simulink model "walkingRobotRL3D"  (R2020b)
settings: Solver=ode23t  StartTime=0.0  StopTime=Tf  RelTol=1e-2  EnableMultiTasking=on
PreLoadFcn:
  | robotParametersRL
undefined symbols (not defined in the file): agent, ankleD_pitch_jointMAX, ankleD_pitch_jointMIN, ankleD_roll_jointMAX, ankleD_roll_jointMIN, ankleI_pitch_jointMAX, ankleI_pitch_jointMIN, ankleI_roll_jointMAX, ankleI_roll_jointMIN, getSampleTime, height_plane, hipD_pitch_jointMAX, hipD_pitch_jointMIN, hipD_roll_jointMAX, hipD_roll_jointMIN, hipI_pitch_jointMAX, hipI_pitch_jointMIN, hipI_roll_jointMAX, hipI_roll_jointMIN, init_angs_L, init_angs_R, init_height, joint_damping, joint_limit_damping, joint_limit_stiffness, joint_stiffness, kneeD_jointMAX, kneeD_jointMIN, kneeI_jointMAX, kneeI_jointMIN, lower_leg_I0, lower_leg_length, lower_leg_mass, lower_leg_x, lower_leg_y, muscle_nominal_length, p10_ankleD_roll, plane_x, plane_y, regulator_type, tau, Tf, torso_height, torso_length, torso_offset_x, torso_offset_z, torso_width, torso_x, torso_y, torso_z, Ts, upper_leg_I0, upper_leg_length, upper_leg_mass, upper_leg_x, upper_leg_y, v10_ankleD_pitch, v10_ankleD_roll, v10_ankleI_pitch, v10_ankleI_roll ... (+41)
libraries: sm_lib x222, simulink x183, nesl_utility x130, walkingRobotUtils x69, rllib x2
(part 10 of 24)

== system walkingRobotRL3D/Check if Done22/Check correct behaviour of the muscles/Subsystem1 ==
  In1 : Inport
  In2 : Inport  Port=2
  Compare To Constant : simulink/Logic and Bit Operations/Compare To Constant  relop=<=  const=v10_ankleD_pitch  OutDataTypeStr=boolean
  Compare To Constant1 : simulink/Logic and Bit Operations/Compare To Constant  relop=>=  const=v20_ankleD_pitch  OutDataTypeStr=boolean
  Compare To Constant2 : simulink/Logic and Bit Operations/Compare To Constant  relop=>=  const=v10_ankleD_pitch  OutDataTypeStr=boolean
  Compare To Constant3 : simulink/Logic and Bit Operations/Compare To Constant  relop=<=  const=v20_ankleD_pitch  OutDataTypeStr=boolean
  Logical Operator : Logic  AllPortsSameDT=off  OutDataTypeStr=boolean
  Logical Operator1 : Logic  AllPortsSameDT=off  OutDataTypeStr=boolean
  OR : Logic  Operator=OR  IconShape=distinctive  AllPortsSameDT=off  OutDataTypeStr=boolean
  Out1 : Outport
  wires:
  In2/1 -> Compare To Constant3/1, Compare To Constant1/1
  Compare To Constant/1 -> Logical Operator/1
  Compare To Constant2/1 -> Logical Operator1/1
  OR/1 -> Out1/1
  Logical Operator1/1 -> OR/2
  In1/1 -> Compare To Constant2/1, Compare To Constant/1
  Logical Operator/1 -> OR/1
  Compare To Constant1/1 -> Logical Operator/2
  Compare To Constant3/1 -> Logical Operator1/2

== system walkingRobotRL3D/Check if Done22/Check correct behaviour of the muscles/Subsystem2 ==
  In1 : Inport
  In2 : Inport  Port=2
  Compare To Constant : simulink/Logic and Bit Operations/Compare To Constant  relop=>=  const=v10_kneeD  OutDataTypeStr=boolean
  Compare To Constant1 : simulink/Logic and Bit Operations/Compare To Constant  relop=<=  const=v20_kneeD/2  OutDataTypeStr=boolean
  Compare To Constant2 : simulink/Logic and Bit Operations/Compare To Constant  relop=>=  const=v20_kneeD/2  OutDataTypeStr=boolean
  Compare To Constant3 : simulink/Logic and Bit Operations/Compare To Constant  relop=<=  const=v20_kneeD  OutDataTypeStr=boolean
  Logical Operator : Logic  AllPortsSameDT=off  OutDataTypeStr=boolean
  Logical Operator1 : Logic  AllPortsSameDT=off  OutDataTypeStr=boolean
  OR : Logic  Operator=OR  IconShape=distinctive  AllPortsSameDT=off  OutDataTypeStr=boolean
  Out1 : Outport
  wires:
  Compare To Constant/1 -> Logical Operator/1
  Compare To Constant2/1 -> Logical Operator1/1
  OR/1 -> Out1/1
  Logical Operator1/1 -> OR/2
  Logical Operator/1 -> OR/1
  Compare To Constant1/1 -> Logical Operator/2
  Compare To Constant3/1 -> Logical Operator1/2
  In1/1 -> Compare To Constant1/1, Compare To Constant/1
  In2/1 -> Compare To Constant3/1, Compare To Constant2/1

== system walkingRobotRL3D/Check if Done22/Check correct behaviour of the muscles/Subsystem3 ==
  In1 : Inport
  In2 : Inport  Port=2
  Compare To Constant : simulink/Logic and Bit Operations/Compare To Constant  relop=<=  const=v10_hipD_roll  OutDataTypeStr=boolean
  Compare To Constant1 : simulink/Logic and Bit Operations/Compare To Constant  relop=>=  const=v20_hipD_roll  OutDataTypeStr=boolean
  Compare To Constant2 : simulink/Logic and Bit Operations/Compare To Constant  relop=>=  const=v10_hipD_roll  OutDataTypeStr=boolean
  Compare To Constant3 : simulink/Logic and Bit Operations/Compare To Constant  relop=<=  const=v20_hipD_roll  OutDataTypeStr=boolean
  Logical Operator : Logic  AllPortsSameDT=off  OutDataTypeStr=boolean
  Logical Operator1 : Logic  AllPortsSameDT=off  OutDataTypeStr=boolean
  OR : Logic  Operator=OR  IconShape=distinctive  AllPortsSameDT=off  OutDataTypeStr=boolean
  Out1 : Outport
  wires:
  In2/1 -> Compare To Constant3/1, Compare To Constant1/1
  Compare To Constant/1 -> Logical Operator/1
  Compare To Constant2/1 -> Logical Operator1/1
  OR/1 -> Out1/1
  Logical Operator1/1 -> OR/2
  In1/1 -> Compare To Constant2/1, Compare To Constant/1
  Logical Operator/1 -> OR/1
  Compare To Constant1/1 -> Logical Operator/2
  Compare To Constant3/1 -> Logical Operator1/2

== system walkingRobotRL3D/Check if Done22/Check correct behaviour of the muscles/Subsystem4 ==
  In1 : Inport
  In2 : Inport  Port=2
  Compare To Constant : simulink/Logic and Bit Operations/Compare To Constant  relop=<=  const=v10_hipD_pitch  OutDataTypeStr=boolean
  Compare To Constant1 : simulink/Logic and Bit Operations/Compare To Constant  relop=>=  const=v20_hipD_pitch  OutDataTypeStr=boolean
  Compare To Constant2 : simulink/Logic and Bit Operations/Compare To Constant  relop=>=  const=v10_hipD_pitch  OutDataTypeStr=boolean
  Compare To Constant3 : simulink/Logic and Bit Operations/Compare To Constant  relop=<=  const=v20_hipD_pitch  OutDataTypeStr=boolean
  Logical Operator : Logic  AllPortsSameDT=off  OutDataTypeStr=boolean
  Logical Operator1 : Logic  AllPortsSameDT=off  OutDataTypeStr=boolean
  OR : Logic  Operator=OR  IconShape=distinctive  AllPortsSameDT=off  OutDataTypeStr=boolean
  Out1 : Outport
  wires:
  In2/1 -> Compare To Constant3/1, Compare To Constant1/1
  Compare To Constant/1 -> Logical Operator/1
  Compare To Constant2/1 -> Logical Operator1/1
  OR/1 -> Out1/1
  Logical Operator1/1 -> OR/2
  In1/1 -> Compare To Constant2/1, Compare To Constant/1
  Logical Operator/1 -> OR/1
  Compare To Constant1/1 -> Logical Operator/2
  Compare To Constant3/1 -> Logical Operator1/2

== system walkingRobotRL3D/Check if Done22/Check correct behaviour of the muscles/Subsystem5 ==
  In1 : Inport
  In2 : Inport  Port=2
  Compare To Constant : simulink/Logic and Bit Operations/Compare To Constant  relop=<=  const=v10_ankleI_roll  OutDataTypeStr=boolean
  Compare To Constant1 : simulink/Logic and Bit Operations/Compare To Constant  relop=>=  const=v20_ankleI_roll  OutDataTypeStr=boolean
  Compare To Constant2 : simulink/Logic and Bit Operations/Compare To Constant  relop=>=  const=v10_ankleI_roll  OutDataTypeStr=boolean
  Compare To Constant3 : simulink/Logic and Bit Operations/Compare To Constant  relop=<=  const=v20_ankleI_roll  OutDataTypeStr=boolean
  Logical Operator : Logic  AllPortsSameDT=off  OutDataTypeStr=boolean
  Logical Operator1 : Logic  AllPortsSameDT=off  OutDataTypeStr=boolean
  OR : Logic  Operator=OR  IconShape=distinctive  AllPortsSameDT=off  OutDataTypeStr=boolean
  Out1 : Outport
  wires:
  In2/1 -> Compare To Constant3/1, Compare To Constant1/1
  Compare To Constant/1 -> Logical Operator/1
  Compare To Constant2/1 -> Logical Operator1/1
  OR/1 -> Out1/1
  Logical Operator1/1 -> OR/2
  In1/1 -> Compare To Constant2/1, Compare To Constant/1
  Logical Operator/1 -> OR/1
  Compare To Constant1/1 -> Logical Operator/2
  Compare To Constant3/1 -> Logical Operator1/2

== system walkingRobotRL3D/Check if Done22/Check correct behaviour of the muscles/Subsystem6 ==
  In1 : Inport
  In2 : Inport  Port=2
  Compare To Constant : simulink/Logic and Bit Operations/Compare To Constant  relop=<=  const=v10_ankleI_pitch  OutDataTypeStr=boolean
  Compare To Constant1 : simulink/Logic and Bit Operations/Compare To Constant  relop=>=  const=v20_ankleI_pitch  OutDataTypeStr=boolean
  Compare To Constant2 : simulink/Logic and Bit Operations/Compare To Constant  relop=>=  const=v10_ankleI_pitch  OutDataTypeStr=boolean
  Compare To Constant3 : simulink/Logic and Bit Operations/Compare To Constant  relop=<=  const=v20_ankleI_pitch  OutDataTypeStr=boolean
  Logical Operator : Logic  AllPortsSameDT=off  OutDataTypeStr=boolean
  Logical Operator1 : Logic  AllPortsSameDT=off  OutDataTypeStr=boolean
  OR : Logic  Operator=OR  IconShape=distinctive  AllPortsSameDT=off  OutDataTypeStr=boolean
  Out1 : Outport
  wires:
  In2/1 -> Compare To Constant3/1, Compare To Constant1/1
  Compare To Constant/1 -> Logical Operator/1
  Compare To Constant2/1 -> Logical Operator1/1
  OR/1 -> Out1/1
  Logical Operator1/1 -> OR/2
  In1/1 -> Compare To Constant2/1, Compare To Constant/1
  Logical Operator/1 -> OR/1
  Compare To Constant1/1 -> Logical Operator/2
  Compare To Constant3/1 -> Logical Operator1/2

== system walkingRobotRL3D/Check if Done22/Check correct behaviour of the muscles/Subsystem7 ==
  In1 : Inport
  In2 : Inport  Port=2
  Compare To Constant : simulink/Logic and Bit Operations/Compare To Constant  relop=<=  const=v10_hipI_roll  OutDataTypeStr=boolean
  Compare To Constant1 : simulink/Logic and Bit Operations/Compare To Constant  relop=>=  const=v20_hipI_roll  OutDataTypeStr=boolean
  Compare To Constant2 : simulink/Logic and Bit Operations/Compare To Constant  relop=>=  const=v10_hipI_roll  OutDataTypeStr=boolean
  Compare To Constant3 : simulink/Logic and Bit Operations/Compare To Constant  relop=<=  const=v20_hipI_roll  OutDataTypeStr=boolean
  Logical Operator : Logic  AllPortsSameDT=off  OutDataTypeStr=boolean
  Logical Operator1 : Logic  AllPortsSameDT=off  OutDataTypeStr=boolean
  OR : Logic  Operator=OR  IconShape=distinctive  AllPortsSameDT=off  OutDataTypeStr=boolean
  Out1 : Outport
  wires:
  In2/1 -> Compare To Constant3/1, Compare To Constant1/1
  Compare To Constant/1 -> Logical Operator/1
  Compare To Constant2/1 -> Logical Operator1/1
  OR/1 -> Out1/1
  Logical Operator1/1 -> OR/2
  In1/1 -> Compare To Constant2/1, Compare To Constant/1
  Logical Operator/1 -> OR/1
  Compare To Constant1/1 -> Logical Operator/2
  Compare To Constant3/1 -> Logical Operator1/2

== system walkingRobotRL3D/Check if Done22/Check correct behaviour of the muscles/Subsystem8 ==
  In1 : Inport
  In2 : Inport  Port=2
  Compare To Constant : simulink/Logic and Bit Operations/Compare To Constant  relop=<=  const=v10_hipI_pitch  OutDataTypeStr=boolean
  Compare To Constant1 : simulink/Logic and Bit Operations/Compare To Constant  relop=>=  const=v20_hipI_pitch  OutDataTypeStr=boolean
  Compare To Constant2 : simulink/Logic and Bit Operations/Compare To Constant  relop=>=  const=v10_hipI_pitch  OutDataTypeStr=boolean
  Compare To Constant3 : simulink/Logic and Bit Operations/Compare To Constant  relop=<=  const=v20_hipI_pitch  OutDataTypeStr=boolean
  Logical Operator : Logic  AllPortsSameDT=off  OutDataTypeStr=boolean
  Logical Operator1 : Logic  AllPortsSameDT=off  OutDataTypeStr=boolean
  OR : Logic  Operator=OR  IconShape=distinctive  AllPortsSameDT=off  OutDataTypeStr=boolean
  Out1 : Outport
  wires:
  In2/1 -> Compare To Constant3/1, Compare To Constant1/1
  Compare To Constant/1 -> Logical Operator/1
  Compare To Constant2/1 -> Logical Operator1/1
  OR/1 -> Out1/1
  Logical Operator1/1 -> OR/2
  In1/1 -> Compare To Constant2/1, Compare To Constant/1
  Logical Operator/1 -> OR/1
  Compare To Constant1/1 -> Logical Operator/2
  Compare To Constant3/1 -> Logical Operator1/2

== system walkingRobotRL3D/Check if Done22/Check correct behaviour of the muscles/Subsystem9 ==
  In1 : Inport
  In2 : Inport  Port=2
  Compare To Constant : simulink/Logic and Bit Operations/Compare To Constant  relop=>=  const=v10_kneeI  OutDataTypeStr=boolean
  Compare To Constant1 : simulink/Logic and Bit Operations/Compare To Constant  relop=<=  const=v20_kneeI/2  OutDataTypeStr=boolean
  Compare To Constant2 : simulink/Logic and Bit Operations/Compare To Constant  relop=>=  const=v20_kneeI/2  OutDataTypeStr=boolean
  Compare To Constant3 : simulink/Logic and Bit Operations/Compare To Constant  relop=<=  const=v20_kneeI  OutDataTypeStr=boolean
  Logical Operator : Logic  AllPortsSameDT=off  OutDataTypeStr=boolean
  Logical Operator1 : Logic  AllPortsSameDT=off  OutDataTypeStr=boolean
  OR : Logic  Operator=OR  IconShape=distinctive  AllPortsSameDT=off  OutDataTypeStr=boolean
  Out1 : Outport
  wires:
  Compare To Constant/1 -> Logical Operator/1
  Compare To Constant2/1 -> Logical Operator1/1
  OR/1 -> Out1/1
  Logical Operator1/1 -> OR/2
  Logical Operator/1 -> OR/1
  Compare To Constant1/1 -> Logical Operator/2
  Compare To Constant3/1 -> Logical Operator1/2
  In1/1 -> Compare To Constant1/1, Compare To Constant/1
  In2/1 -> Compare To Constant3/1, Compare To Constant2/1

== system walkingRobotRL3D/Check if Done3/Check correct behaviour of the muscles/Subsystem ==
  In1 : Inport
  In2 : Inport  Port=2
  Compare To Constant : simulink/Logic and Bit Operations/Compare To Constant  relop=<=  const=v10_ankleD_roll  OutDataTypeStr=boolean
  Compare To Constant1 : simulink/Logic and Bit Operations/Compare To Constant  relop=>=  const=v20_ankleD_roll  OutDataTypeStr=boolean
  Compare To Constant2 : simulink/Logic and Bit Operations/Compare To Constant  relop=>=  const=v10_ankleD_roll  OutDataTypeStr=boolean
  Compare To Constant3 : simulink/Logic and Bit Operations/Compare To Constant  relop=<=  const=v20_ankleD_roll  OutDataTypeStr=boolean
  Logical Operator : Logic  AllPortsSameDT=off  OutDataTypeStr=boolean
  Logical Operator1 : Logic  AllPortsSameDT=off  OutDataTypeStr=boolean
  OR : Logic  Operator=OR  IconShape=distinctive  AllPortsSameDT=off  OutDataTypeStr=boolean
  Out1 : Outport
  wires:
  In2/1 -> Compare To Constant3/1, Compare To Constant1/1
  Compare To Constant/1 -> Logical Operator/1
  Compare To Constant2/1 -> Logical Operator1/1
  OR/1 -> Out1/1
  Logical Operator1/1 -> OR/2
  In1/1 -> Compare To Constant2/1, Compare To Constant/1
  Logical Operator/1 -> OR/1
  Compare To Constant1/1 -> Logical Operator/2
  Compare To Constant3/1 -> Logical Operator1/2

== system walkingRobotRL3D/Check if Done3/Check correct behaviour of the muscles/Subsystem1 ==
  In1 : Inport
  In2 : Inport  Port=2
  Compare To Constant : simulink/Logic and Bit Operations/Compare To Constant  relop=<=  const=v10_ankleD_pitch  OutDataTypeStr=boolean
  Compare To Constant1 : simulink/Logic and Bit Operations/Compare To Constant  relop=>=  const=v20_ankleD_pitch  OutDataTypeStr=boolean
  Compare To Constant2 : simulink/Logic and Bit Operations/Compare To Constant  relop=>=  const=v10_ankleD_pitch  OutDataTypeStr=boolean
  Compare To Constant3 : simulink/Logic and Bit Operations/Compare To Constant  relop=<=  const=v20_ankleD_pitch  OutDataTypeStr=boolean
  Logical Operator : Logic  AllPortsSameDT=off  OutDataTypeStr=boolean
  Logical Operator1 : Logic  AllPortsSameDT=off  OutDataTypeStr=boolean
  OR : Logic  Operator=OR  IconShape=distinctive  AllPortsSameDT=off  OutDataTypeStr=boolean
  Out1 : Outport
  wires:
  In2/1 -> Compare To Constant3/1, Compare To Constant1/1
  Compare To Constant/1 -> Logical Operator/1
  Compare To Constant2/1 -> Logical Operator1/1
  OR/1 -> Out1/1
  Logical Operator1/1 -> OR/2
  In1/1 -> Compare To Constant2/1, Compare To Constant/1
  Logical Operator/1 -> OR/1
  Compare To Constant1/1 -> Logical Operator/2
  Compare To Constant3/1 -> Logical Operator1/2

== system walkingRobotRL3D/Check if Done3/Check correct behaviour of the muscles/Subsystem2 ==
  In1 : Inport
  In2 : Inport  Port=2
  Compare To Constant : simulink/Logic and Bit Operations/Compare To Constant  relop=>=  const=v10_kneeD  OutDataTypeStr=boolean
  Compare To Constant1 : simulink/Logic and Bit Operations/Compare To Constant  relop=<=  const=v20_kneeD/2  OutDataTypeStr=boolean
  Compare To Constant2 : simulink/Logic and Bit Operations/Compare To Constant  relop=>=  const=v20_kneeD/2  OutDataTypeStr=boolean
  Compare To Constant3 : simulink/Logic and Bit Operations/Compare To Constant  relop=<=  const=v20_kneeD  OutDataTypeStr=boolean
  Logical Operator : Logic  AllPortsSameDT=off  OutDataTypeStr=boolean
  Logical Operator1 : Logic  AllPortsSameDT=off  OutDataTypeStr=boolean
  OR : Logic  Operator=OR  IconShape=distinctive  AllPortsSameDT=off  OutDataTypeStr=boolean
  Out1 : Outport
  wires:
  Compare To Constant/1 -> Logical Operator/1
  Compare To Constant2/1 -> Logical Operator1/1
  OR/1 -> Out1/1
  Logical Operator1/1 -> OR/2
  Logical Operator/1 -> OR/1
  Compare To Constant1/1 -> Logical Operator/2
  Compare To Constant3/1 -> Logical Operator1/2
  In1/1 -> Compare To Constant1/1, Compare To Constant/1
  In2/1 -> Compare To Constant3/1, Compare To Constant2/1

== system walkingRobotRL3D/Check if Done3/Check correct behaviour of the muscles/Subsystem3 ==
  In1 : Inport
  In2 : Inport  Port=2
  Compare To Constant : simulink/Logic and Bit Operations/Compare To Constant  relop=<=  const=v10_hipD_roll  OutDataTypeStr=boolean
  Compare To Constant1 : simulink/Logic and Bit Operations/Compare To Constant  relop=>=  const=v20_hipD_roll  OutDataTypeStr=boolean
  Compare To Constant2 : simulink/Logic and Bit Operations/Compare To Constant  relop=>=  const=v10_hipD_roll  OutDataTypeStr=boolean
  Compare To Constant3 : simulink/Logic and Bit Operations/Compare To Constant  relop=<=  const=v20_hipD_roll  OutDataTypeStr=boolean
  Logical Operator : Logic  AllPortsSameDT=off  OutDataTypeStr=boolean
  Logical Operator1 : Logic  AllPortsSameDT=off  OutDataTypeStr=boolean
  OR : Logic  Operator=OR  IconShape=distinctive  AllPortsSameDT=off  OutDataTypeStr=boolean
  Out1 : Outport
  wires:
  In2/1 -> Compare To Constant3/1, Compare To Constant1/1
  Compare To Constant/1 -> Logical Operator/1
  Compare To Constant2/1 -> Logical Operator1/1
  OR/1 -> Out1/1
  Logical Operator1/1 -> OR/2
  In1/1 -> Compare To Constant2/1, Compare To Constant/1
  Logical Operator/1 -> OR/1
  Compare To Constant1/1 -> Logical Operator/2
  Compare To Constant3/1 -> Logical Operator1/2

== system walkingRobotRL3D/Check if Done3/Check correct behaviour of the muscles/Subsystem4 ==
  In1 : Inport
  In2 : Inport  Port=2
  Compare To Constant : simulink/Logic and Bit Operations/Compare To Constant  relop=<=  const=v10_hipD_pitch  OutDataTypeStr=boolean
  Compare To Constant1 : simulink/Logic and Bit Operations/Compare To Constant  relop=>=  const=v20_hipD_pitch  OutDataTypeStr=boolean
  Compare To Constant2 : simulink/Logic and Bit Operations/Compare To Constant  relop=>=  const=v10_hipD_pitch  OutDataTypeStr=boolean
  Compare To Constant3 : simulink/Logic and Bit Operations/Compare To Constant  relop=<=  const=v20_hipD_pitch  OutDataTypeStr=boolean
  Logical Operator : Logic  AllPortsSameDT=off  OutDataTypeStr=boolean
  Logical Operator1 : Logic  AllPortsSameDT=off  OutDataTypeStr=boolean
  OR : Logic  Operator=OR  IconShape=distinctive  AllPortsSameDT=off  OutDataTypeStr=boolean
  Out1 : Outport
  wires:
  In2/1 -> Compare To Constant3/1, Compare To Constant1/1
  Compare To Constant/1 -> Logical Operator/1
  Compare To Constant2/1 -> Logical Operator1/1
  OR/1 -> Out1/1
  Logical Operator1/1 -> OR/2
  In1/1 -> Compare To Constant2/1, Compare To Constant/1
  Logical Operator/1 -> OR/1
  Compare To Constant1/1 -> Logical Operator/2
  Compare To Constant3/1 -> Logical Operator1/2

== system walkingRobotRL3D/Check if Done3/Check correct behaviour of the muscles/Subsystem5 ==
  In1 : Inport
  In2 : Inport  Port=2
  Compare To Constant : simulink/Logic and Bit Operations/Compare To Constant  relop=<=  const=v10_ankleI_roll  OutDataTypeStr=boolean
  Compare To Constant1 : simulink/Logic and Bit Operations/Compare To Constant  relop=>=  const=v20_ankleI_roll  OutDataTypeStr=boolean
  Compare To Constant2 : simulink/Logic and Bit Operations/Compare To Constant  relop=>=  const=v10_ankleI_roll  OutDataTypeStr=boolean
  Compare To Constant3 : simulink/Logic and Bit Operations/Compare To Constant  relop=<=  const=v20_ankleI_roll  OutDataTypeStr=boolean
  Logical Operator : Logic  AllPortsSameDT=off  OutDataTypeStr=boolean
  Logical Operator1 : Logic  AllPortsSameDT=off  OutDataTypeStr=boolean
  OR : Logic  Operator=OR  IconShape=distinctive  AllPortsSameDT=off  OutDataTypeStr=boolean
  Out1 : Outport
  wires:
  In2/1 -> Compare To Constant3/1, Compare To Constant1/1
  Compare To Constant/1 -> Logical Operator/1
  Compare To Constant2/1 -> Logical Operator1/1
  OR/1 -> Out1/1
  Logical Operator1/1 -> OR/2
  In1/1 -> Compare To Constant2/1, Compare To Constant/1
  Logical Operator/1 -> OR/1
  Compare To Constant1/1 -> Logical Operator/2
  Compare To Constant3/1 -> Logical Operator1/2

== system walkingRobotRL3D/Check if Done3/Check correct behaviour of the muscles/Subsystem6 ==
  In1 : Inport
  In2 : Inport  Port=2
  Compare To Constant : simulink/Logic and Bit Operations/Compare To Constant  relop=<=  const=v10_ankleI_pitch  OutDataTypeStr=boolean
  Compare To Constant1 : simulink/Logic and Bit Operations/Compare To Constant  relop=>=  const=v20_ankleI_pitch  OutDataTypeStr=boolean
  Compare To Constant2 : simulink/Logic and Bit Operations/Compare To Constant  relop=>=  const=v10_ankleI_pitch  OutDataTypeStr=boolean
  Compare To Constant3 : simulink/Logic and Bit Operations/Compare To Constant  relop=<=  const=v20_ankleI_pitch  OutDataTypeStr=boolean
  Logical Operator : Logic  AllPortsSameDT=off  OutDataTypeStr=boolean
  Logical Operator1 : Logic  AllPortsSameDT=off  OutDataTypeStr=boolean
  OR : Logic  Operator=OR  IconShape=distinctive  AllPortsSameDT=off  OutDataTypeStr=boolean
  Out1 : Outport
  wires:
  In2/1 -> Compare To Constant3/1, Compare To Constant1/1
  Compare To Constant/1 -> Logical Operator/1
  Compare To Constant2/1 -> Logical Operator1/1
  OR/1 -> Out1/1
  Logical Operator1/1 -> OR/2
  In1/1 -> Compare To Constant2/1, Compare To Constant/1
  Logical Operator/1 -> OR/1
  Compare To Constant1/1 -> Logical Operator/2
  Compare To Constant3/1 -> Logical Operator1/2

== system walkingRobotRL3D/Check if Done3/Check correct behaviour of the muscles/Subsystem7 ==
  In1 : Inport
  In2 : Inport  Port=2
  Compare To Constant : simulink/Logic and Bit Operations/Compare To Constant  relop=<=  const=v10_hipI_roll  OutDataTypeStr=boolean
  Compare To Constant1 : simulink/Logic and Bit Operations/Compare To Constant  relop=>=  const=v20_hipI_roll  OutDataTypeStr=boolean
  Compare To Constant2 : simulink/Logic and Bit Operations/Compare To Constant  relop=>=  const=v10_hipI_roll  OutDataTypeStr=boolean
  Compare To Constant3 : simulink/Logic and Bit Operations/Compare To Constant  relop=<=  const=v20_hipI_roll  OutDataTypeStr=boolean
  Logical Operator : Logic  AllPortsSameDT=off  OutDataTypeStr=boolean
  Logical Operator1 : Logic  AllPortsSameDT=off  OutDataTypeStr=boolean
  OR : Logic  Operator=OR  IconShape=distinctive  AllPortsSameDT=off  OutDataTypeStr=boolean
  Out1 : Outport
  wires:
  In2/1 -> Compare To Constant3/1, Compare To Constant1/1
  Compare To Constant/1 -> Logical Operator/1
  Compare To Constant2/1 -> Logical Operator1/1
  OR/1 -> Out1/1
  Logical Operator1/1 -> OR/2
  In1/1 -> Compare To Constant2/1, Compare To Constant/1
  Logical Operator/1 -> OR/1
  Compare To Constant1/1 -> Logical Operator/2
  Compare To Constant3/1 -> Logical Operator1/2

== system walkingRobotRL3D/Check if Done3/Check correct behaviour of the muscles/Subsystem8 ==
  In1 : Inport
  In2 : Inport  Port=2
  Compare To Constant : simulink/Logic and Bit Operations/Compare To Constant  relop=<=  const=v10_hipI_pitch  OutDataTypeStr=boolean
  Compare To Constant1 : simulink/Logic and Bit Operations/Compare To Constant  relop=>=  const=v20_hipI_pitch  OutDataTypeStr=boolean
  Compare To Constant2 : simulink/Logic and Bit Operations/Compare To Constant  relop=>=  const=v10_hipI_pitch  OutDataTypeStr=boolean
  Compare To Constant3 : simulink/Logic and Bit Operations/Compare To Constant  relop=<=  const=v20_hipI_pitch  OutDataTypeStr=boolean
  Logical Operator : Logic  AllPortsSameDT=off  OutDataTypeStr=boolean
  Logical Operator1 : Logic  AllPortsSameDT=off  OutDataTypeStr=boolean
  OR : Logic  Operator=OR  IconShape=distinctive  AllPortsSameDT=off  OutDataTypeStr=boolean
  Out1 : Outport
  wires:
  In2/1 -> Compare To Constant3/1, Compare To Constant1/1
  Compare To Constant/1 -> Logical Operator/1
  Compare To Constant2/1 -> Logical Operator1/1
  OR/1 -> Out1/1
  Logical Operator1/1 -> OR/2
  In1/1 -> Compare To Constant2/1, Compare To Constant/1
  Logical Operator/1 -> OR/1
  Compare To Constant1/1 -> Logical Operator/2
  Compare To Constant3/1 -> Logical Operator1/2

== system walkingRobotRL3D/Check if Done3/Check correct behaviour of the muscles/Subsystem9 ==
  In1 : Inport
  In2 : Inport  Port=2
  Compare To Constant : simulink/Logic and Bit Operations/Compare To Constant  relop=>=  const=v10_kneeI  OutDataTypeStr=boolean
  Compare To Constant1 : simulink/Logic and Bit Operations/Compare To Constant  relop=<=  const=v20_kneeI/2  OutDataTypeStr=boolean
  Compare To Constant2 : simulink/Logic and Bit Operations/Compare To Constant  relop=>=  const=v20_kneeI/2  OutDataTypeStr=boolean
  Compare To Constant3 : simulink/Logic and Bit Operations/Compare To Constant  relop=<=  const=v20_kneeI  OutDataTypeStr=boolean
  Logical Operator : Logic  AllPortsSameDT=off  OutDataTypeStr=boolean
  Logical Operator1 : Logic  AllPortsSameDT=off  OutDataTypeStr=boolean
  OR : Logic  Operator=OR  IconShape=distinctive  AllPortsSameDT=off  OutDataTypeStr=boolean
  Out1 : Outport
  wires:
  Compare To Constant/1 -> Logical Operator/1
  Compare To Constant2/1 -> Logical Operator1/1
  OR/1 -> Out1/1
  Logical Operator1/1 -> OR/2
  Logical Operator/1 -> OR/1
  Compare To Constant1/1 -> Logical Operator/2
  Compare To Constant3/1 -> Logical Operator1/2
  In1/1 -> Compare To Constant1/1, Compare To Constant/1
  In2/1 -> Compare To Constant3/1, Compare To Constant2/1

== system walkingRobotRL3D/RL Agent3/accumulate_reward/cumsum ==
  rwd : Inport
  Enable : EnablePort
  Sum : Sum  Inputs=|++
  Unit Delay : UnitDelay  SampleTime=-1  HasFrameUpgradeWarning=on
  cumulative_rwd : Outport  VectorParamsAs1DForOutWhenUnconnected=off
  wires:
  Unit Delay/1 -> Sum/2
  Sum/1 -> cumulative_rwd/1, Unit Delay/1
  rwd/1 -> Sum/1

== system walkingRobotRL3D/RL Agent33/accumulate_reward/cumsum ==
  rwd : Inport
  Enable : EnablePort
  Sum : Sum  Inputs=|++
  Unit Delay : UnitDelay  SampleTime=-1  HasFrameUpgradeWarning=on
  cumulative_rwd : Outport  VectorParamsAs1DForOutWhenUnconnected=off
  wires:
  Unit Delay/1 -> Sum/2
  Sum/1 -> cumulative_rwd/1, Unit Delay/1
  rwd/1 -> Sum/1

== system walkingRobotRL3D/Walking Robot/DYNAMIC MODEL OF PAM FOR LEFT LEG/Dynamic Model Antagonisitic PAM1 ==
  V1 : Inport
  V2 : Inport  Port=2
  Abs : Abs  Commented=through
  Constant : Constant
  Constant1 : Constant
  F(x,P) mode (Muscles 1) : MATLAB Function  TreatAsAtomicUnit=on
  F(x,P) mode (Muscles 1)1 : MATLAB Function  TreatAsAtomicUnit=on
  Proportional Regulator (Muscles 1) : MATLAB Function  TreatAsAtomicUnit=on
  Proportional Regulator (Muscles 2) : MATLAB Function  TreatAsAtomicUnit=on
  Spring and damping model : Subsystem
  F1 : Outport
  F2 : Outport  Port=2
  wires:
  Constant1/1 -> Proportional Regulator (Muscles 2)/2(reg_type)
  F(x,P) mode (Muscles 1)/1(F1) -> Spring and damping model/1(F1), F1/1
  Proportional Regulator (Muscles 2)/1(p1) -> Spring and damping model/4(P2), F(x,P) mode (Muscles 1)1/1(P2)
  Proportional Regulator (Muscles 1)/1(p1) -> Spring and damping model/3(P1), F(x,P) mode (Muscles 1)/1(P1)
  Spring and damping model/1(x2) -> F(x,P) mode (Muscles 1)1/2(x_muscle2)
  F(x,P) mode (Muscles 1)1/1(F2) -> Abs/1
  Constant/1 -> Proportional Regulator (Muscles 1)/2(reg_type)
  V2/1 -> Proportional Regulator (Muscles 2)/1(V1)
  V1/1 -> Proportional Regulator (Muscles 1)/1(V1)
  Abs/1 -> F2/1, Spring and damping model/2(F2)
  Spring and damping model/2(x1) -> F(x,P) mode (Muscles 1)/2(x_muscle1)

== system walkingRobotRL3D/Walking Robot/DYNAMIC MODEL OF PAM FOR LEFT LEG/Dynamic Model Antagonisitic PAM2 ==
  V1 : Inport
  V2 : Inport  Port=2
  Abs : Abs  Commented=through
  Constant : Constant
  Constant1 : Constant
  F(x,P) mode (Muscles 1) : MATLAB Function  TreatAsAtomicUnit=on
  F(x,P) mode (Muscles 1)1 : MATLAB Function  TreatAsAtomicUnit=on
  Proportional Regulator (Muscles 1) : MATLAB Function  TreatAsAtomicUnit=on
  Proportional Regulator (Muscles 2) : MATLAB Function  TreatAsAtomicUnit=on
  Spring and damping model : Subsystem
  F1 : Outport
  F2 : Outport  Port=2
  wires:
  Constant1/1 -> Proportional Regulator (Muscles 2)/2(reg_type)
  F(x,P) mode (Muscles 1)/1(F1) -> Spring and damping model/1(F1), F1/1
  Proportional Regulator (Muscles 2)/1(p1) -> Spring and damping model/4(P2), F(x,P) mode (Muscles 1)1/1(P2)
  Proportional Regulator (Muscles 1)/1(p1) -> Spring and damping model/3(P1), F(x,P) mode (Muscles 1)/1(P1)
  Spring and damping model/1(x2) -> F(x,P) mode (Muscles 1)1/2(x_muscle2)
  F(x,P) mode (Muscles 1)1/1(F2) -> Abs/1
  Constant/1 -> Proportional Regulator (Muscles 1)/2(reg_type)
  V2/1 -> Proportional Regulator (Muscles 2)/1(V1)
  V1/1 -> Proportional Regulator (Muscles 1)/1(V1)
  Abs/1 -> F2/1, Spring and damping model/2(F2)
  Spring and damping model/2(x1) -> F(x,P) mode (Muscles 1)/2(x_muscle1)

== system walkingRobotRL3D/Walking Robot/DYNAMIC MODEL OF PAM FOR LEFT LEG/Dynamic Model Antagonisitic PAM3 ==
  V1 : Inport
  V2 : Inport  Port=2
  Abs : Abs  Commented=through
  Constant : Constant
  Constant1 : Constant
  F(x,P) mode (Muscles 1) : MATLAB Function  TreatAsAtomicUnit=on
  F(x,P) mode (Muscles 1)1 : MATLAB Function  TreatAsAtomicUnit=on
  Proportional Regulator (Muscles 1) : MATLAB Function  TreatAsAtomicUnit=on
  Proportional Regulator (Muscles 2) : MATLAB Function  TreatAsAtomicUnit=on
  Spring and damping model : Subsystem
  F1 : Outport
  F2 : Outport  Port=2
  wires:
  Constant1/1 -> Proportional Regulator (Muscles 2)/2(reg_type)
  F(x,P) mode (Muscles 1)/1(F1) -> Spring and damping model/1(F1), F1/1
  Proportional Regulator (Muscles 2)/1(p1) -> Spring and damping model/4(P2), F(x,P) mode (Muscles 1)1/1(P2)
  Proportional Regulator (Muscles 1)/1(p1) -> Spring and damping model/3(P1), F(x,P) mode (Muscles 1)/1(P1)
  Spring and damping model/1(x2) -> F(x,P) mode (Muscles 1)1/2(x_muscle2)
  F(x,P) mode (Muscles 1)1/1(F2) -> Abs/1
  Constant/1 -> Proportional Regulator (Muscles 1)/2(reg_type)
  V2/1 -> Proportional Regulator (Muscles 2)/1(V1)
  V1/1 -> Proportional Regulator (Muscles 1)/1(V1)
  Abs/1 -> F2/1, Spring and damping model/2(F2)
  Spring and damping model/2(x1) -> F(x,P) mode (Muscles 1)/2(x_muscle1)

== system walkingRobotRL3D/Walking Robot/DYNAMIC MODEL OF PAM FOR LEFT LEG/Dynamic Model Antagonisitic PAM4 ==
  V1 : Inport
  V2 : Inport  Port=2
  Abs : Abs  Commented=through
  Constant : Constant
  Constant1 : Constant
  F(x,P) mode (Muscles 1) : MATLAB Function  TreatAsAtomicUnit=on
  F(x,P) mode (Muscles 1)1 : MATLAB Function  TreatAsAtomicUnit=on
  Proportional Regulator (Muscles 1) : MATLAB Function  TreatAsAtomicUnit=on
  Proportional Regulator (Muscles 2) : MATLAB Function  TreatAsAtomicUnit=on
  Spring and damping model : Subsystem
  F1 : Outport
  F2 : Outport  Port=2
  wires:
  Constant1/1 -> Proportional Regulator (Muscles 2)/2(reg_type)
  F(x,P) mode (Muscles 1)/1(F1) -> Spring and damping model/1(F1), F1/1
  Proportional Regulator (Muscles 2)/1(p1) -> Spring and damping model/4(P2), F(x,P) mode (Muscles 1)1/1(P2)
  Proportional Regulator (Muscles 1)/1(p1) -> Spring and damping model/3(P1), F(x,P) mode (Muscles 1)/1(P1)
  Spring and damping model/1(x2) -> F(x,P) mode (Muscles 1)1/2(x_muscle2)
  F(x,P) mode (Muscles 1)1/1(F2) -> Abs/1
  Constant/1 -> Proportional Regulator (Muscles 1)/2(reg_type)
  V2/1 -> Proportional Regulator (Muscles 2)/1(V1)
  V1/1 -> Proportional Regulator (Muscles 1)/1(V1)
  Abs/1 -> F2/1, Spring and damping model/2(F2)
  Spring and damping model/2(x1) -> F(x,P) mode (Muscles 1)/2(x_muscle1)

== system walkingRobotRL3D/Walking Robot/DYNAMIC MODEL OF PAM FOR LEFT LEG/Dynamic Model Antagonisitic PAM5 ==
  V1 : Inport
  V2 : Inport  Port=2
  Abs : Abs  Commented=through
  Constant : Constant
  Constant1 : Constant
  F(x,P) mode (Muscles 1) : MATLAB Function  TreatAsAtomicUnit=on
  F(x,P) mode (Muscles 1)1 : MATLAB Function  TreatAsAtomicUnit=on
  Proportional Regulator (Muscles 1) : MATLAB Function  TreatAsAtomicUnit=on
  Proportional Regulator (Muscles 2) : MATLAB Function  TreatAsAtomicUnit=on
  Spring and damping model : Subsystem
  F1 : Outport
  F2 : Outport  Port=2
  wires:
  Constant1/1 -> Proportional Regulator (Muscles 2)/2(reg_type)
  F(x,P) mode (Muscles 1)/1(F1) -> Spring and damping model/1(F1), F1/1
  Proportional Regulator (Muscles 2)/1(p1) -> Spring and damping model/4(P2), F(x,P) mode (Muscles 1)1/1(P2)
  Proportional Regulator (Muscles 1)/1(p1) -> Spring and damping model/3(P1), F(x,P) mode (Muscles 1)/1(P1)
  Spring and damping model/1(x2) -> F(x,P) mode (Muscles 1)1/2(x_muscle2)
  F(x,P) mode (Muscles 1)1/1(F2) -> Abs/1
  Constant/1 -> Proportional Regulator (Muscles 1)/2(reg_type)
  V2/1 -> Proportional Regulator (Muscles 2)/1(V1)
  V1/1 -> Proportional Regulator (Muscles 1)/1(V1)
  Abs/1 -> F2/1, Spring and damping model/2(F2)
  Spring and damping model/2(x1) -> F(x,P) mode (Muscles 1)/2(x_muscle1)

== system walkingRobotRL3D/Walking Robot/DYNAMIC MODEL OF PAM FOR RIGHT LEG/Dynamic Model Antagonisitic PAM1 ==
  V1 : Inport
  V2 : Inport  Port=2
  Abs : Abs  Commented=through
  Constant : Constant
  Constant1 : Constant
  F(x,P) mode (Muscles 1) : MATLAB Function  TreatAsAtomicUnit=on
  F(x,P) mode (Muscles 1)1 : MATLAB Function  TreatAsAtomicUnit=on
  Proportional Regulator (Muscles 1) : MATLAB Function  TreatAsAtomicUnit=on
  Proportional Regulator (Muscles 2) : MATLAB Function  TreatAsAtomicUnit=on
  Spring and damping model : Subsystem
  F1 : Outport
  F2 : Outport  Port=2
  wires:
  Constant1/1 -> Proportional Regulator (Muscles 2)/2(reg_type)
  F(x,P) mode (Muscles 1)/1(F1) -> Spring and damping model/1(F1), F1/1
  Proportional Regulator (Muscles 2)/1(p1) -> Spring and damping model/4(P2), F(x,P) mode (Muscles 1)1/1(P2)
  Proportional Regulator (Muscles 1)/1(p1) -> Spring and damping model/3(P1), F(x,P) mode (Muscles 1)/1(P1)
  Spring and damping model/1(x2) -> F(x,P) mode (Muscles 1)1/2(x_muscle2)
  F(x,P) mode (Muscles 1)1/1(F2) -> Abs/1
  Constant/1 -> Proportional Regulator (Muscles 1)/2(reg_type)
  V2/1 -> Proportional Regulator (Muscles 2)/1(V1)
  V1/1 -> Proportional Regulator (Muscles 1)/1(V1)
  Abs/1 -> F2/1, Spring and damping model/2(F2)
  Spring and damping model/2(x1) -> F(x,P) mode (Muscles 1)/2(x_muscle1)

== system walkingRobotRL3D/Walking Robot/DYNAMIC MODEL OF PAM FOR RIGHT LEG/Dynamic Model Antagonisitic PAM2 ==
  V1 : Inport
  V2 : Inport  Port=2
  Abs : Abs  Commented=through
  Constant : Constant
  Constant1 : Constant
  F(x,P) mode (Muscles 1) : MATLAB Function  TreatAsAtomicUnit=on
  F(x,P) mode (Muscles 1)1 : MATLAB Function  TreatAsAtomicUnit=on
  Proportional Regulator (Muscles 1) : MATLAB Function  TreatAsAtomicUnit=on
  Proportional Regulator (Muscles 2) : MATLAB Function  TreatAsAtomicUnit=on
  Spring and damping model : Subsystem
  F1 : Outport
  F2 : Outport  Port=2
  wires:
  Constant1/1 -> Proportional Regulator (Muscles 2)/2(reg_type)
  F(x,P) mode (Muscles 1)/1(F1) -> Spring and damping model/1(F1), F1/1
  Proportional Regulator (Muscles 2)/1(p1) -> Spring and damping model/4(P2), F(x,P) mode (Muscles 1)1/1(P2)
  Proportional Regulator (Muscles 1)/1(p1) -> Spring and damping model/3(P1), F(x,P) mode (Muscles 1)/1(P1)
  Spring and damping model/1(x2) -> F(x,P) mode (Muscles 1)1/2(x_muscle2)
  F(x,P) mode (Muscles 1)1/1(F2) -> Abs/1
  Constant/1 -> Proportional Regulator (Muscles 1)/2(reg_type)
  V2/1 -> Proportional Regulator (Muscles 2)/1(V1)
  V1/1 -> Proportional Regulator (Muscles 1)/1(V1)
  Abs/1 -> F2/1, Spring and damping model/2(F2)
  Spring and damping model/2(x1) -> F(x,P) mode (Muscles 1)/2(x_muscle1)

== system walkingRobotRL3D/Walking Robot/DYNAMIC MODEL OF PAM FOR RIGHT LEG/Dynamic Model Antagonisitic PAM3 ==
  V1 : Inport
  V2 : Inport  Port=2
  Abs : Abs  Commented=through
  Constant : Constant
  Constant1 : Constant
  F(x,P) mode (Muscles 1) : MATLAB Function  TreatAsAtomicUnit=on
  F(x,P) mode (Muscles 1)1 : MATLAB Function  TreatAsAtomicUnit=on
  Proportional Regulator (Muscles 1) : MATLAB Function  TreatAsAtomicUnit=on
  Proportional Regulator (Muscles 2) : MATLAB Function  TreatAsAtomicUnit=on
  Spring and damping model : Subsystem
  F1 : Outport
  F2 : Outport  Port=2
  wires:
  Constant1/1 -> Proportional Regulator (Muscles 2)/2(reg_type)
  F(x,P) mode (Muscles 1)/1(F1) -> Spring and damping model/1(F1), F1/1
  Proportional Regulator (Muscles 2)/1(p1) -> Spring and damping model/4(P2), F(x,P) mode (Muscles 1)1/1(P2)
  Proportional Regulator (Muscles 1)/1(p1) -> Spring and damping model/3(P1), F(x,P) mode (Muscles 1)/1(P1)
  Spring and damping model/1(x2) -> F(x,P) mode (Muscles 1)1/2(x_muscle2)
  F(x,P) mode (Muscles 1)1/1(F2) -> Abs/1
  Constant/1 -> Proportional Regulator (Muscles 1)/2(reg_type)
  V2/1 -> Proportional Regulator (Muscles 2)/1(V1)
  V1/1 -> Proportional Regulator (Muscles 1)/1(V1)
  Abs/1 -> F2/1, Spring and damping model/2(F2)
  Spring and damping model/2(x1) -> F(x,P) mode (Muscles 1)/2(x_muscle1)

== system walkingRobotRL3D/Walking Robot/DYNAMIC MODEL OF PAM FOR RIGHT LEG/Dynamic Model Antagonisitic PAM4 ==
  V1 : Inport
  V2 : Inport  Port=2
  Abs : Abs  Commented=through
  Constant : Constant
  Constant1 : Constant
  F(x,P) mode (Muscles 1) : MATLAB Function  TreatAsAtomicUnit=on
  F(x,P) mode (Muscles 1)1 : MATLAB Function  TreatAsAtomicUnit=on
  Proportional Regulator (Muscles 1) : MATLAB Function  TreatAsAtomicUnit=on
  Proportional Regulator (Muscles 2) : MATLAB Function  TreatAsAtomicUnit=on
  Spring and damping model : Subsystem
  F1 : Outport
  F2 : Outport  Port=2
  wires:
  Constant1/1 -> Proportional Regulator (Muscles 2)/2(reg_type)
  F(x,P) mode (Muscles 1)/1(F1) -> Spring and damping model/1(F1), F1/1
  Proportional Regulator (Muscles 2)/1(p1) -> Spring and damping model/4(P2), F(x,P) mode (Muscles 1)1/1(P2)
  Proportional Regulator (Muscles 1)/1(p1) -> Spring and damping model/3(P1), F(x,P) mode (Muscles 1)/1(P1)
  Spring and damping model/1(x2) -> F(x,P) mode (Muscles 1)1/2(x_muscle2)
  F(x,P) mode (Muscles 1)1/1(F2) -> Abs/1
  Constant/1 -> Proportional Regulator (Muscles 1)/2(reg_type)
  V2/1 -> Proportional Regulator (Muscles 2)/1(V1)
  V1/1 -> Proportional Regulator (Muscles 1)/1(V1)
  Abs/1 -> F2/1, Spring and damping model/2(F2)
  Spring and damping model/2(x1) -> F(x,P) mode (Muscles 1)/2(x_muscle1)

== system walkingRobotRL3D/Walking Robot/DYNAMIC MODEL OF PAM FOR RIGHT LEG/Dynamic Model Antagonisitic PAM5 ==
  V1 : Inport
  V2 : Inport  Port=2
  Abs : Abs  Commented=through
  Constant : Constant
  Constant1 : Constant
  F(x,P) mode (Muscles 1) : MATLAB Function  TreatAsAtomicUnit=on
  F(x,P) mode (Muscles 1)1 : MATLAB Function  TreatAsAtomicUnit=on
  Proportional Regulator (Muscles 1) : MATLAB Function  TreatAsAtomicUnit=on
  Proportional Regulator (Muscles 2) : MATLAB Function  TreatAsAtomicUnit=on
  Spring and damping model : Subsystem
  F1 : Outport
  F2 : Outport  Port=2
  wires:
  Constant1/1 -> Proportional Regulator (Muscles 2)/2(reg_type)
  F(x,P) mode (Muscles 1)/1(F1) -> Spring and damping model/1(F1), F1/1
  Proportional Regulator (Muscles 2)/1(p1) -> Spring and damping model/4(P2), F(x,P) mode (Muscles 1)1/1(P2)
  Proportional Regulator (Muscles 1)/1(p1) -> Spring and damping model/3(P1), F(x,P) mode (Muscles 1)/1(P1)
  Spring and damping model/1(x2) -> F(x,P) mode (Muscles 1)1/2(x_muscle2)
  F(x,P) mode (Muscles 1)1/1(F2) -> Abs/1
  Constant/1 -> Proportional Regulator (Muscles 1)/2(reg_type)
  V2/1 -> Proportional Regulator (Muscles 2)/1(V1)
  V1/1 -> Proportional Regulator (Muscles 1)/1(V1)
  Abs/1 -> F2/1, Spring and damping model/2(F2)
  Spring and damping model/2(x1) -> F(x,P) mode (Muscles 1)/2(x_muscle1)

== system walkingRobotRL3D/Walking Robot/Sensors/Calculate Actuator Power 3D ==
  meas : Inport
  Add : Sum  Inputs=5
  Bus Selector : BusSelector  OutputSignals=ankle_roll_angle,ankle_roll_speed,ankle_pitch_angle,ankle_pitch_speed,knee_angle,knee_speed,hip_roll_angle,hip_roll_speed,hip_pitch_angle,hip_pitch_speed
  Product{,1..4} (5 alike) : Product
  P : Outport  VectorParamsAs1DForOutWhenUnconnected=off
  wires:
  meas/1 -> Bus Selector/1
  Product2/1 -> Add/4
  Product1/1 -> Add/2
  Product/1 -> Add/1
  Add/1 -> P/1
  Bus Selector/1 -> Product/1  "<ankle_roll_angle>"
  Bus Selector/2 -> Product/2  "<ankle_roll_speed>"
  Bus Selector/3 -> Product1/1  "<ankle_pitch_angle>"
  Bus Selector/4 -> Product1/2  "<ankle_pitch_speed>"
  Bus Selector/5 -> Product3/1  "<knee_angle>"
  Bus Selector/6 -> Product3/2  "<knee_speed>"
  Bus Selector/7 -> Product2/1  "<hip_roll_angle>"
  Bus Selector/8 -> Product2/2  "<hip_roll_speed>"
  Bus Selector/10 -> Product4/2  "<hip_pitch_speed>"
  Bus Selector/9 -> Product4/1  "<hip_pitch_angle>"
  Product4/1 -> Add/5
  Product3/1 -> Add/3

== system walkingRobotRL3D/Walking Robot/Sensors/Calculate Actuator Power 3D1 ==
  meas : Inport
  Add : Sum  Inputs=5
  Bus Selector : BusSelector  OutputSignals=ankle_roll_angle,ankle_roll_speed,ankle_pitch_angle,ankle_pitch_speed,knee_angle,knee_speed,hip_roll_angle,hip_roll_speed,hip_pitch_angle,hip_pitch_speed
  Product{,1..4} (5 alike) : Product
  P : Outport  VectorParamsAs1DForOutWhenUnconnected=off
  wires:
  Product3/1 -> Add/3
  Product4/1 -> Add/5
  Bus Selector/9 -> Product4/1  "<hip_pitch_angle>"
  Bus Selector/10 -> Product4/2  "<hip_pitch_speed>"
  Bus Selector/8 -> Product2/2  "<hip_roll_speed>"
  Bus Selector/7 -> Product2/1  "<hip_roll_angle>"
  Bus Selector/6 -> Product3/2  "<knee_speed>"
  Bus Selector/5 -> Product3/1  "<knee_angle>"
  Bus Selector/4 -> Product1/2  "<ankle_pitch_speed>"
  Bus Selector/3 -> Product1/1  "<ankle_pitch_angle>"
  Bus Selector/2 -> Product/2  "<ankle_roll_speed>"
  Bus Selector/1 -> Product/1  "<ankle_roll_angle>"
  Add/1 -> P/1
  Product/1 -> Add/1
  Product1/1 -> Add/2
  Product2/1 -> Add/4
  meas/1 -> Bus Selector/1

== system walkingRobotRL3D/Walking Robot (Angle based)/Antagonistic PAM Left Leg/ankleI_pitch PAM ==
  V1 : Inport
  V2 : Inport  Port=2
  Constant : Constant
  Constant1 : Constant
  F(x,P) mode (Muscles 1) : MATLAB Function  TreatAsAtomicUnit=on
  F(x,P) mode (Muscles 1)1 : MATLAB Function  TreatAsAtomicUnit=on
  Proportional Regulator (Muscles 1) : MATLAB Function  TreatAsAtomicUnit=on
  Proportional Regulator (Muscles 2) : MATLAB Function  TreatAsAtomicUnit=on
  Spring and damping model : Subsystem
  F1 : Outport
  F2 : Outport  Port=2
  x1 : Outport  Port=3
  x2 : Outport  Port=4
  wires:
  Constant1/1 -> Proportional Regulator (Muscles 2)/2(reg_type)
  F(x,P) mode (Muscles 1)/1(F1) -> F1/1, Spring and damping model/1(F1)
  Proportional Regulator (Muscles 2)/1(p1) -> Spring and damping model/4(P2), F(x,P) mode (Muscles 1)1/1(P2)
  Proportional Regulator (Muscles 1)/1(p1) -> Spring and damping model/3(P1), F(x,P) mode (Muscles 1)/1(P1)
  Spring and damping model/2(x2) -> x2/1, F(x,P) mode (Muscles 1)1/2(x_muscle2)
  Spring and damping model/1(x1) -> x1/1, F(x,P) mode (Muscles 1)/2(x_muscle1)
  F(x,P) mode (Muscles 1)1/1(F2) -> F2/1, Spring and damping model/2(F2)
  Constant/1 -> Proportional Regulator (Muscles 1)/2(reg_type)
  V2/1 -> Proportional Regulator (Muscles 2)/1(V1)
  V1/1 -> Proportional Regulator (Muscles 1)/1(V1)

== system walkingRobotRL3D/Walking Robot (Angle based)/Antagonistic PAM Left Leg/ankleI_roll PAM ==
  V1 : Inport
  V2 : Inport  Port=2
  Constant : Constant
  Constant1 : Constant
  F(x,P) mode (Muscles 1) : MATLAB Function  TreatAsAtomicUnit=on
  F(x,P) mode (Muscles 1)1 : MATLAB Function  TreatAsAtomicUnit=on
  Proportional Regulator (Muscles 1) : MATLAB Function  TreatAsAtomicUnit=on
  Proportional Regulator (Muscles 2) : MATLAB Function  TreatAsAtomicUnit=on
  Spring and damping model : Subsystem
  F1 : Outport
  F2 : Outport  Port=2
  x1 : Outport  Port=3
  x2 : Outport  Port=4
  wires:
  Constant1/1 -> Proportional Regulator (Muscles 2)/2(reg_type)
  F(x,P) mode (Muscles 1)/1(F1) -> F1/1, Spring and damping model/1(F1)
  Proportional Regulator (Muscles 2)/1(p1) -> Spring and damping model/4(P2), F(x,P) mode (Muscles 1)1/1(P2)
  Proportional Regulator (Muscles 1)/1(p1) -> Spring and damping model/3(P1), F(x,P) mode (Muscles 1)/1(P1)
  Spring and damping model/2(x2) -> x2/1, F(x,P) mode (Muscles 1)1/2(x_muscle2)
  Spring and damping model/1(x1) -> x1/1, F(x,P) mode (Muscles 1)/2(x_muscle1)
  F(x,P) mode (Muscles 1)1/1(F2) -> F2/1, Spring and damping model/2(F2)
  Constant/1 -> Proportional Regulator (Muscles 1)/2(reg_type)
  V2/1 -> Proportional Regulator (Muscles 2)/1(V1)
  V1/1 -> Proportional Regulator (Muscles 1)/1(V1)

== system walkingRobotRL3D/Walking Robot (Angle based)/Antagonistic PAM Left Leg/hipI_pitch PAM ==
  V1 : Inport
  V2 : Inport  Port=2
  Constant : Constant
  Constant1 : Constant
  F(x,P) mode (Muscles 1) : MATLAB Function  TreatAsAtomicUnit=on
  F(x,P) mode (Muscles 1)1 : MATLAB Function  TreatAsAtomicUnit=on
  Proportional Regulator (Muscles 1) : MATLAB Function  TreatAsAtomicUnit=on
  Proportional Regulator (Muscles 2) : MATLAB Function  TreatAsAtomicUnit=on
  Spring and damping model : Subsystem
  F1 : Outport
  F2 : Outport  Port=2
  x1 : Outport  Port=3
  x2 : Outport  Port=4
  wires:
  Constant1/1 -> Proportional Regulator (Muscles 2)/2(reg_type)
  F(x,P) mode (Muscles 1)/1(F1) -> F1/1, Spring and damping model/1(F1)
  Proportional Regulator (Muscles 2)/1(p1) -> Spring and damping model/4(P2), F(x,P) mode (Muscles 1)1/1(P2)
  Proportional Regulator (Muscles 1)/1(p1) -> Spring and damping model/3(P1), F(x,P) mode (Muscles 1)/1(P1)
  Spring and damping model/2(x2) -> x2/1, F(x,P) mode (Muscles 1)1/2(x_muscle2)
  Spring and damping model/1(x1) -> x1/1, F(x,P) mode (Muscles 1)/2(x_muscle1)
  F(x,P) mode (Muscles 1)1/1(F2) -> F2/1, Spring and damping model/2(F2)
  Constant/1 -> Proportional Regulator (Muscles 1)/2(reg_type)
  V2/1 -> Proportional Regulator (Muscles 2)/1(V1)
  V1/1 -> Proportional Regulator (Muscles 1)/1(V1)

== system walkingRobotRL3D/Walking Robot (Angle based)/Antagonistic PAM Left Leg/hipI_roll PAM ==
  V1 : Inport
  V2 : Inport  Port=2
  Constant : Constant
  Constant1 : Constant
  F(x,P) mode (Muscles 1) : MATLAB Function  TreatAsAtomicUnit=on
  F(x,P) mode (Muscles 1)1 : MATLAB Function  TreatAsAtomicUnit=on
  Proportional Regulator (Muscles 1) : MATLAB Function  TreatAsAtomicUnit=on
  Proportional Regulator (Muscles 2) : MATLAB Function  TreatAsAtomicUnit=on
  Spring and damping model : Subsystem
  F1 : Outport
  F2 : Outport  Port=2
  x1 : Outport  Port=3
  x2 : Outport  Port=4
  wires:
  Constant1/1 -> Proportional Regulator (Muscles 2)/2(reg_type)
  F(x,P) mode (Muscles 1)/1(F1) -> F1/1, Spring and damping model/1(F1)
  Proportional Regulator (Muscles 2)/1(p1) -> Spring and damping model/4(P2), F(x,P) mode (Muscles 1)1/1(P2)
  Proportional Regulator (Muscles 1)/1(p1) -> Spring and damping model/3(P1), F(x,P) mode (Muscles 1)/1(P1)
  Spring and damping model/2(x2) -> x2/1, F(x,P) mode (Muscles 1)1/2(x_muscle2)
  Spring and damping model/1(x1) -> x1/1, F(x,P) mode (Muscles 1)/2(x_muscle1)
  F(x,P) mode (Muscles 1)1/1(F2) -> F2/1, Spring and damping model/2(F2)
  Constant/1 -> Proportional Regulator (Muscles 1)/2(reg_type)
  V2/1 -> Proportional Regulator (Muscles 2)/1(V1)
  V1/1 -> Proportional Regulator (Muscles 1)/1(V1)

== system walkingRobotRL3D/Walking Robot (Angle based)/Antagonistic PAM Left Leg/kneeI PAM ==
  V1 : Inport
  V2 : Inport  Port=2
  Constant : Constant
  Constant1 : Constant
  F(x,P) mode (Muscles 1) : MATLAB Function  TreatAsAtomicUnit=on
  F(x,P) mode (Muscles 1)1 : MATLAB Function  TreatAsAtomicUnit=on
  Proportional Regulator (Muscles 1) : MATLAB Function  TreatAsAtomicUnit=on
  Proportional Regulator (Muscles 2) : MATLAB Function  TreatAsAtomicUnit=on
  Spring and damping model : Subsystem
  F1 : Outport
  F2 : Outport  Port=2
  x1 : Outport  Port=3
  x2 : Outport  Port=4
  wires:
  Constant1/1 -> Proportional Regulator (Muscles 2)/2(reg_type)
  F(x,P) mode (Muscles 1)/1(F1) -> F1/1, Spring and damping model/1(F1)
  Proportional Regulator (Muscles 2)/1(p1) -> Spring and damping model/4(P2), F(x,P) mode (Muscles 1)1/1(P2)
  Proportional Regulator (Muscles 1)/1(p1) -> Spring and damping model/3(P1), F(x,P) mode (Muscles 1)/1(P1)
  Spring and damping model/2(x2) -> x2/1, F(x,P) mode (Muscles 1)1/2(x_muscle2)
  Spring and damping model/1(x1) -> x1/1, F(x,P) mode (Muscles 1)/2(x_muscle1)
  F(x,P) mode (Muscles 1)1/1(F2) -> F2/1, Spring and damping model/2(F2)
  Constant/1 -> Proportional Regulator (Muscles 1)/2(reg_type)
  V2/1 -> Proportional Regulator (Muscles 2)/1(V1)
  V1/1 -> Proportional Regulator (Muscles 1)/1(V1)
